simulink model "FinalSimulinkBlock"  (R2017b)
settings: Solver=FixedStepAuto  StartTime=0.0  StopTime=inf  RelTol=1e-3  EnableMultiTasking=on
libraries: simulink_extras x6, simulink x2, embdlinuxlib x2
settings Model: SimulationMode=external  Creator=gtsia  LastModifiedBy=DELL 5548
settings SolverCC: PositivePriorityOrder=on
settings OptimizationCC: PassReuseOutputArgsAs=Individual arguments  MaxStackSize=64
settings DebuggingCC: ParameterTunabilityLossMsg=error
settings HardwareCC: ProdBitPerPointer=32  ProdBitPerSizeT=32  ProdBitPerPtrDiffT=32  ProdLargestAtomicInteger=Long  ProdLargestAtomicFloat=Double  ProdWordSize=32  ProdHWDeviceType=ARM Compatible->ARM Cortex
settings SFSimCC: MATLABDynamicMemAlloc=off
settings RTWCC: SystemTargetFile=ert.tlc  HardwareBoard=Raspberry Pi  TemplateMakefile=ert_default_tmf  GenerateReport=on  Toolchain=GNU GCC Raspberry Pi  IncludeHyperlinkInReport=on  LaunchReport=on  GenerateTraceInfo=on  GenerateTraceReport=on  GenerateTraceReportSl=on  GenerateTraceReportSf=on  GenerateTraceReportEml=on
settings CodeAppCC: ForceParamTrailComments=on  IgnoreCustomStorageClasses=off  OperatorAnnotations=on  SimulinkDataObjDesc=on  SFDataObjDesc=on  InsertBlockDesc=on
settings ERTTargetCC: SupportContinuousTime=on  SupportVariableSizeSignals=on

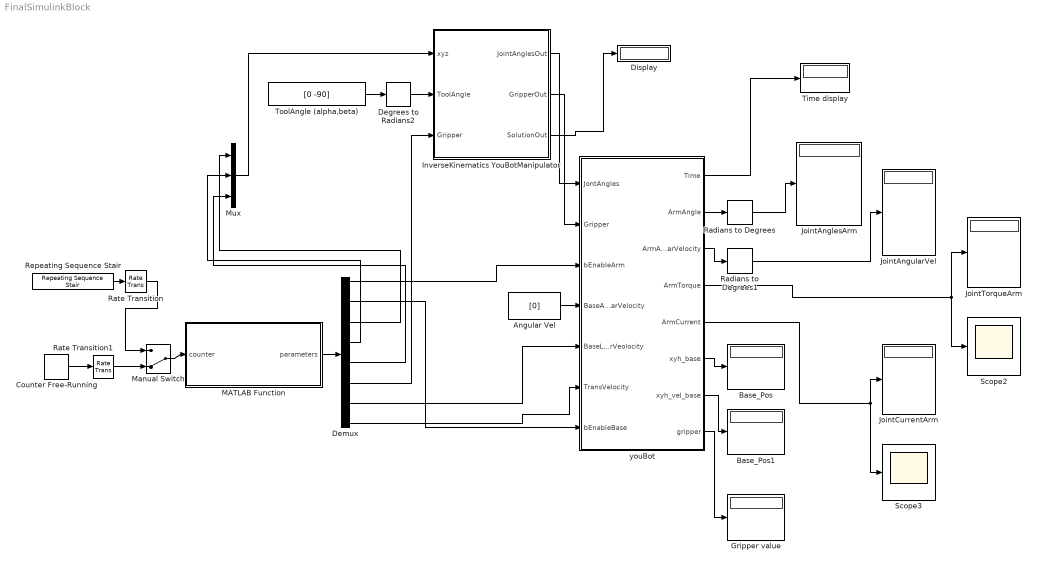
== system FinalSimulinkBlock ==
  Angular Vel : Constant  Value=[0]
  Base_Pos : Display
  Base_Pos1 : Display
  Counter Free-Running : simulink/Sources/Counter Free-Running  NumBits=8  tsamp=6
  Degrees to Radians2 : simulink_extras/Transformations/Degrees to Radians
  Demux : Demux  Outputs=8
  Display : Display
  Gripper value : Display
  InverseKinematics YouBotManipulator : Subsystem
  JointAnglesArm : Display
  JointAngularVel : Display
  JointCurrentArm : Display
  "JointTorqueArm " : Display
  MATLAB Function : MATLAB Function  TreatAsAtomicUnit=on
  Manual Switch : ManualSwitch  CurrentSetting=0
  Mux : Mux  Inputs=3
  Radians to Degrees : simulink_extras/Transformations/Radians to Degrees
  Radians to Degrees1 : simulink_extras/Transformations/Radians to Degrees
  Rate Transition : RateTransition
  Rate Transition1 : RateTransition
  Repeating Sequence Stair : simulink/Sources/Repeating Sequence Stair  OutValues=[0 1 2 3 4 5 6 7 8 9 10 11 11 11 11 11 11].'  tsamp=6  OutMin=[]  OutMax=[]  OutDataTypeStr=double  OutputDataTypeScalingMode=double  OutDataType=fixdt(0,8)  ConRadixGroup=Best Precision: Vector-wise  OutScaling=2^-12
  Scope2 : Scope
  Scope3 : Scope
  Time display : Display
  ToolAngle (alpha,beta) : Constant  Value=[0 -90]
  "youBot " : Subsystem  TreatAsAtomicUnit=on
  wires:
  InverseKinematics YouBotManipulator/2("GripperOut ") -> "youBot "/2(Gripper)
  "youBot "/3(ArmAngularVelocity) -> Radians to Degrees1/1
  "youBot "/1(Time) -> Time display/1
  Radians to Degrees1/1 -> JointAngularVel/1
  Radians to Degrees/1 -> JointAnglesArm/1
  "youBot "/2(ArmAngle) -> Radians to Degrees/1
  "youBot "/6(xyh_base) -> Base_Pos/1
  "youBot "/7(xyh_vel_base) -> Base_Pos1/1
  InverseKinematics YouBotManipulator/1(JointAnglesOut) -> "youBot "/1(JontAngles)
  ToolAngle (alpha,beta)/1 -> Degrees to Radians2/1
  Degrees to Radians2/1 -> InverseKinematics YouBotManipulator/2(ToolAngle)
  Demux/1 -> "youBot "/3(bEnableArm)
  Demux/2 -> "youBot "/7(bEnableBase)
  Demux/3 -> Mux/1
  Demux/4 -> Mux/2
  Demux/5 -> Mux/3
  Demux/6 -> InverseKinematics YouBotManipulator/3(Gripper)
  Demux/7 -> "youBot "/5(BaseLinearVeolocity)
  Demux/8 -> "youBot "/6(TransVelocity)
  Repeating Sequence Stair/1 -> Rate Transition/1
  Manual Switch/1 -> MATLAB Function/1(counter)
  Counter Free-Running/1 -> Rate Transition1/1
  Rate Transition/1 -> Manual Switch/1
  Rate Transition1/1 -> Manual Switch/2
  MATLAB Function/1(parameters) -> Demux/1
  Mux/1 -> InverseKinematics YouBotManipulator/1("xyz ")
  "youBot "/8(gripper) -> Gripper value/1
  InverseKinematics YouBotManipulator/3(SolutionOut) -> Display/1
  Angular Vel/1 -> "youBot "/4("BaseAngularVelocity ")
  "youBot "/4(ArmTorque) -> "JointTorqueArm "/1, Scope2/1
  "youBot "/5(ArmCurrent) -> Scope3/1, JointCurrentArm/1

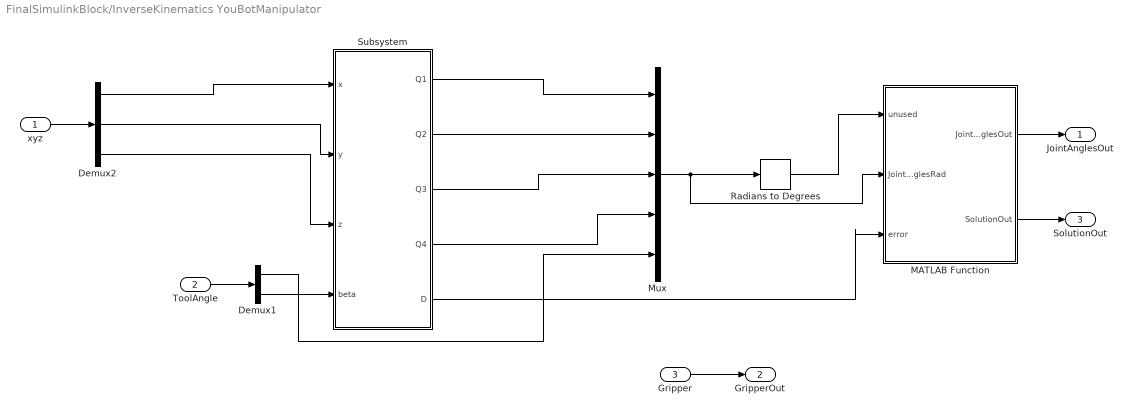
== system FinalSimulinkBlock/InverseKinematics YouBotManipulator ==
  "xyz " : Inport
  ToolAngle : Inport  Port=2
  Gripper : Inport  Port=3
  Demux1 : Demux  Outputs=2
  Demux2 : Demux  Outputs=3
  MATLAB Function : MATLAB Function  TreatAsAtomicUnit=on
  Mux : Mux  Inputs=5
  Radians to Degrees : simulink_extras/Transformations/Radians to Degrees
  Subsystem : Subsystem
  JointAnglesOut : Outport
  "GripperOut " : Outport  Port=2
  SolutionOut : Outport  Port=3
  wires:
  Subsystem/5(D) -> MATLAB Function/3(error)
  Mux/1 -> MATLAB Function/2(JointAnglesRad), Radians to Degrees/1
  Demux1/1 -> Mux/5
  Demux1/2 -> Subsystem/4(beta)
  ToolAngle/1 -> Demux1/1
  "xyz "/1 -> Demux2/1
  Subsystem/3(Q3) -> Mux/3
  Subsystem/2(Q2) -> Mux/2
  Radians to Degrees/1 -> MATLAB Function/1(unused)
  Subsystem/4(Q4) -> Mux/4
  Demux2/1 -> Subsystem/1(x)
  Demux2/2 -> Subsystem/2(y)
  Demux2/3 -> Subsystem/3(z)
  Subsystem/1(Q1) -> Mux/1
  MATLAB Function/2(SolutionOut) -> SolutionOut/1
  MATLAB Function/1(JointAnglesOut) -> JointAnglesOut/1
  Gripper/1 -> "GripperOut "/1

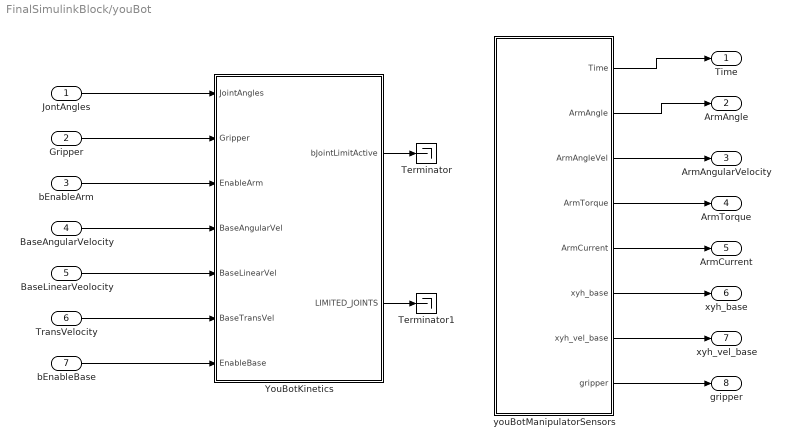
== system FinalSimulinkBlock/youBot  ==
  JontAngles : Inport
  Gripper : Inport  Port=2
  bEnableArm : Inport  Port=3
  "BaseAngularVelocity " : Inport  Port=4
  BaseLinearVeolocity : Inport  Port=5
  TransVelocity : Inport  Port=6
  bEnableBase : Inport  Port=7
  Terminator : Terminator
  Terminator1 : Terminator
  "YouBotKinetics " : Subsystem
  youBotManipulatorSensors : Subsystem
  Time : Outport
  ArmAngle : Outport  Port=2
  ArmAngularVelocity : Outport  Port=3
  ArmTorque : Outport  Port=4
  ArmCurrent : Outport  Port=5
  xyh_base : Outport  Port=6
  xyh_vel_base : Outport  Port=7
  gripper : Outport  Port=8
  wires:
  JontAngles/1 -> "YouBotKinetics "/1(JointAngles)
  Gripper/1 -> "YouBotKinetics "/2(Gripper)
  bEnableArm/1 -> "YouBotKinetics "/3(EnableArm)
  "BaseAngularVelocity "/1 -> "YouBotKinetics "/4(BaseAngularVel)
  BaseLinearVeolocity/1 -> "YouBotKinetics "/5(BaseLinearVel)
  bEnableBase/1 -> "YouBotKinetics "/7("EnableBase ")
  TransVelocity/1 -> "YouBotKinetics "/6(BaseTransVel)
  youBotManipulatorSensors/1(Time) -> Time/1
  youBotManipulatorSensors/2(ArmAngle) -> ArmAngle/1
  youBotManipulatorSensors/3(ArmAngleVel) -> ArmAngularVelocity/1
  youBotManipulatorSensors/4(ArmTorque) -> ArmTorque/1
  youBotManipulatorSensors/5("ArmCurrent ") -> ArmCurrent/1
  youBotManipulatorSensors/6(xyh_base) -> xyh_base/1
  youBotManipulatorSensors/7(xyh_vel_base) -> xyh_vel_base/1
  youBotManipulatorSensors/8(gripper) -> gripper/1
  "YouBotKinetics "/1(bJointLimitActive) -> Terminator/1
  "YouBotKinetics "/2("LIMITED_JOINTS ") -> Terminator1/1

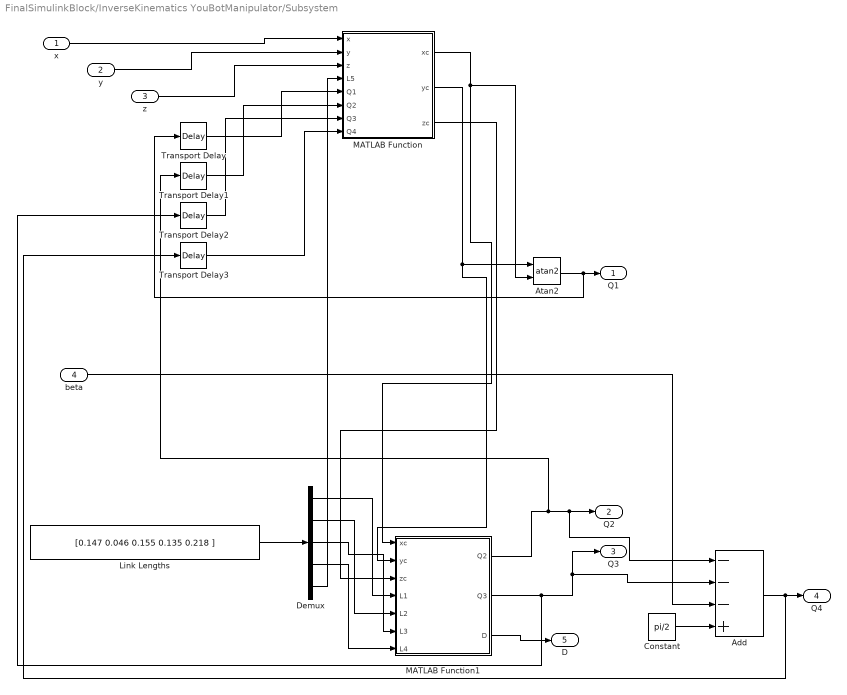
== system FinalSimulinkBlock/InverseKinematics YouBotManipulator/Subsystem ==
  x : Inport
  y : Inport  Port=2
  z : Inport  Port=3
  beta : Inport  Port=4
  Add : Sum  Inputs=---+
  Atan2 : Trigonometry  Operator=atan2
  Constant : Constant  Value=pi/2
  Demux : Demux  Outputs=5
  Link Lengths : Constant  Value=[0.147 0.046 0.155 0.135 0.218 ]
  MATLAB Function : MATLAB Function  TreatAsAtomicUnit=on
  MATLAB Function1 : MATLAB Function  TreatAsAtomicUnit=on
  Transport Delay{,1..3} (4 alike) : TransportDelay
  Q1 : Outport
  Q2 : Outport  Port=2
  Q3 : Outport  Port=3
  Q4 : Outport  Port=4
  D : Outport  Port=5
  wires:
  Demux/2 -> MATLAB Function1/5(L2)
  MATLAB Function/1(xc) -> Atan2/2, MATLAB Function1/1(xc)
  x/1 -> MATLAB Function/1(x)
  z/1 -> MATLAB Function/3(z)
  MATLAB Function1/1(Q2) -> Transport Delay1/1, Q2/1, Add/1
  Add/1 -> Transport Delay3/1, Q4/1
  y/1 -> MATLAB Function/2(y)
  MATLAB Function/3(zc) -> MATLAB Function1/3(zc)
  Link Lengths/1 -> Demux/1
  Demux/4 -> MATLAB Function1/7(L4)
  MATLAB Function1/3(D) -> D/1
  Constant/1 -> Add/4
  MATLAB Function/2(yc) -> Atan2/1, MATLAB Function1/2(yc)
  MATLAB Function1/2(Q3) -> Transport Delay2/1, Q3/1, Add/2
  Demux/3 -> MATLAB Function1/6(L3)
  Demux/1 -> MATLAB Function1/4(L1)
  Atan2/1 -> Transport Delay/1, Q1/1
  beta/1 -> Add/3
  Demux/5 -> MATLAB Function/4(L5)
  Transport Delay/1 -> MATLAB Function/5(Q1)
  Transport Delay1/1 -> MATLAB Function/6(Q2)
  Transport Delay2/1 -> MATLAB Function/7(Q3)
  Transport Delay3/1 -> MATLAB Function/8(Q4)

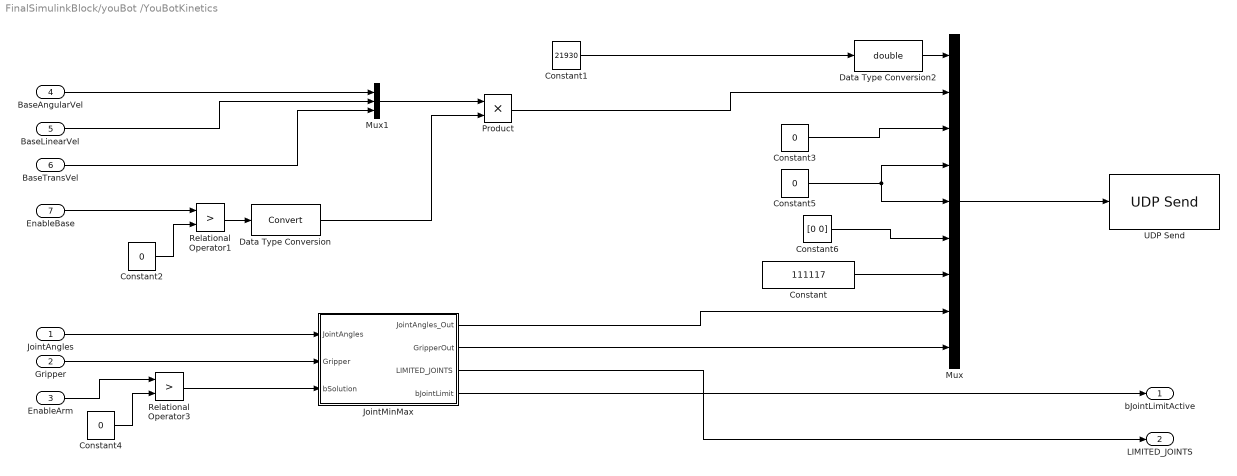
== system FinalSimulinkBlock/youBot /YouBotKinetics  ==
  JointAngles : Inport
  Gripper : Inport  Port=2
  EnableArm : Inport  Port=3
  BaseAngularVel : Inport  Port=4
  BaseLinearVel : Inport  Port=5
  BaseTransVel : Inport  Port=6
  "EnableBase " : Inport  Port=7
  Constant : Constant  Value=111117
  Constant1 : Constant  Value=21930
  Constant{2..5} (4 alike) : Constant  Value=0
  Constant6 : Constant  Value=[0 0]
  Data Type Conversion : DataTypeConversion
  Data Type Conversion2 : DataTypeConversion  OutDataTypeStr=double
  JointMinMax : Subsystem
  Mux : Mux  Inputs=[1 3 1 1 1 2 1 5 1]
  Mux1 : Mux  Inputs=[1 1 1]
  Product : Product
  Relational Operator1 : RelationalOperator  Operator=>  OutDataTypeStr=boolean  RndMeth=Nearest
  Relational Operator3 : RelationalOperator  Operator=>  OutDataTypeStr=boolean  RndMeth=Nearest
  UDP Send : embdlinuxlib/UDP Send  remoteURL='192.168.0.2'  remotePort=25005  localURL='255.255.255.255'  localPortSource=Automatically determine  localPort=-1  sampletime=-1  blockPlatform=Raspberry Pi  separateLengthPort=0
      settings: SourceProductName=Simulink Support Package for Raspberry Pi Hardware  SourceProductBaseCode=RASPPI
  bJointLimitActive : Outport
  "LIMITED_JOINTS " : Outport  Port=2
  wires:
  Mux/1 -> UDP Send/1
  Data Type Conversion2/1 -> Mux/1
  Constant1/1 -> Data Type Conversion2/1
  JointMinMax/1(JointAngles_Out) -> Mux/8
  JointMinMax/2(GripperOut) -> Mux/9
  Gripper/1 -> JointMinMax/2(Gripper)
  JointAngles/1 -> JointMinMax/1(JointAngles)
  JointMinMax/3("LIMITED_JOINTS ") -> "LIMITED_JOINTS "/1
  JointMinMax/4("bJointLimit ") -> bJointLimitActive/1
  Constant/1 -> Mux/7
  BaseAngularVel/1 -> Mux1/1
  BaseLinearVel/1 -> Mux1/2
  BaseTransVel/1 -> Mux1/3
  Constant2/1 -> Relational Operator1/2
  "EnableBase "/1 -> Relational Operator1/1
  Mux1/1 -> Product/1
  Relational Operator1/1 -> Data Type Conversion/1
  Data Type Conversion/1 -> Product/2
  Product/1 -> Mux/2
  Constant4/1 -> Relational Operator3/2
  EnableArm/1 -> Relational Operator3/1
  Constant3/1 -> Mux/3
  Constant5/1 -> Mux/5, Mux/4
  Constant6/1 -> Mux/6
  Relational Operator3/1 -> JointMinMax/3(bSolution)

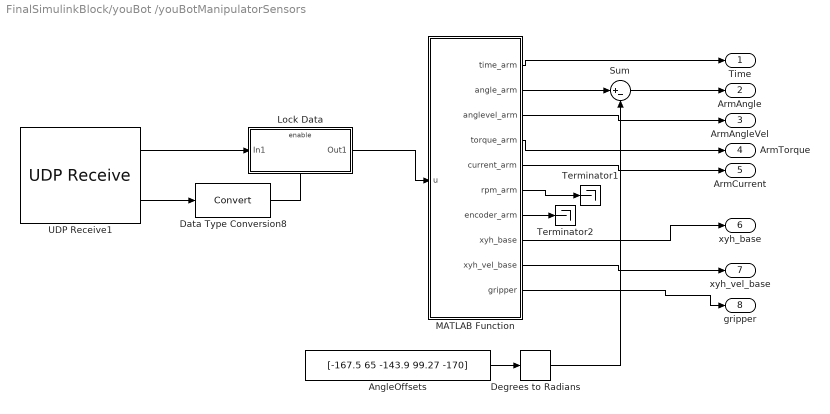
== system FinalSimulinkBlock/youBot /youBotManipulatorSensors ==
  AngleOffsets : Constant  Value=[-167.5 65 -143.9 99.27 -170]
  Data Type Conversion8 : DataTypeConversion
  Degrees to Radians : simulink_extras/Transformations/Degrees to Radians
  Lock Data : Subsystem  TreatAsAtomicUnit=on
  MATLAB Function : MATLAB Function  TreatAsAtomicUnit=on
  Sum : Sum  Inputs=|+-
  Terminator1 : Terminator
  Terminator2 : Terminator
  UDP Receive1 : embdlinuxlib/UDP Receive  localURL='0.0.0.0'  localPort=25611  remoteURL='0.0.0.0'  remotePort=-1  recvBufferSize=8192  signalDatatype=double  dims=62  isVarSize=off  showBlockingTime=off  blockingTime=0  sampletime=0.05  blockPlatform=Raspberry Pi
      settings: SourceProductName=Simulink Support Package for Raspberry Pi Hardware  SourceProductBaseCode=RASPPI
  Time : Outport
  ArmAngle : Outport  Port=2
  ArmAngleVel : Outport  Port=3
  ArmTorque : Outport  Port=4
  "ArmCurrent " : Outport  Port=5
  xyh_base : Outport  Port=6
  xyh_vel_base : Outport  Port=7
  gripper : Outport  Port=8
  wires:
  UDP Receive1/1 -> Lock Data/1(In1)
  Lock Data/1(Out1) -> MATLAB Function/1(u)
  Data Type Conversion8/1 -> Lock Data/Enable
  UDP Receive1/2 -> Data Type Conversion8/1
  MATLAB Function/1(time_arm) -> Time/1
  MATLAB Function/3(anglevel_arm) -> ArmAngleVel/1
  MATLAB Function/4(torque_arm) -> ArmTorque/1
  MATLAB Function/5(current_arm) -> "ArmCurrent "/1
  AngleOffsets/1 -> Degrees to Radians/1
  Sum/1 -> ArmAngle/1
  MATLAB Function/2(angle_arm) -> Sum/1
  Degrees to Radians/1 -> Sum/2
  MATLAB Function/8(xyh_base) -> xyh_base/1
  MATLAB Function/9(xyh_vel_base) -> xyh_vel_base/1
  MATLAB Function/10(gripper) -> gripper/1
  MATLAB Function/6(rpm_arm) -> Terminator1/1
  MATLAB Function/7(encoder_arm) -> Terminator2/1

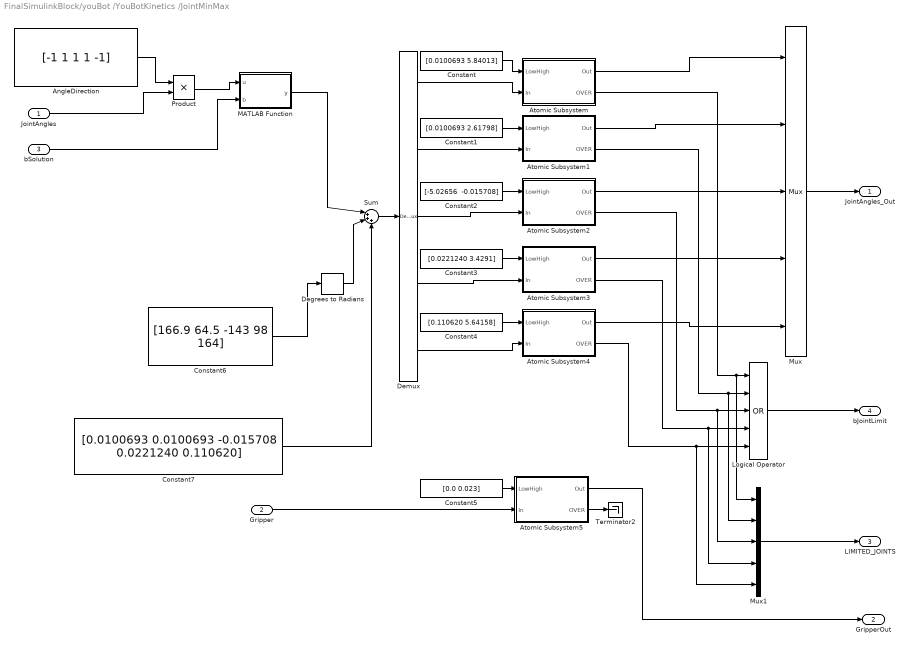
== system FinalSimulinkBlock/youBot /YouBotKinetics /JointMinMax ==
  JointAngles : Inport
  Gripper : Inport  Port=2
  bSolution : Inport  Port=3
  AngleDirection : Constant  Value=[-1 1 1 1 -1]
  Atomic Subsystem : Subsystem  TreatAsAtomicUnit=on
  Atomic Subsystem1 : Subsystem  TreatAsAtomicUnit=on
  Atomic Subsystem2 : Subsystem  TreatAsAtomicUnit=on
  Atomic Subsystem3 : Subsystem  TreatAsAtomicUnit=on
  Atomic Subsystem4 : Subsystem  TreatAsAtomicUnit=on
  Atomic Subsystem5 : Subsystem  TreatAsAtomicUnit=on
  Constant : Constant  Value=[0.0100693 5.84013]
  Constant1 : Constant  Value=[0.0100693 2.61798]
  Constant2 : Constant  Value="[-5.02656  -0.015708]"
  Constant3 : Constant  Value=[0.0221240 3.4291]
  Constant4 : Constant  Value=[0.110620 5.64158]
  Constant5 : Constant  Value=[0.0 0.023]
  Constant6 : Constant  Value=[166.9 64.5 -143 98 164]
  Constant7 : Constant  Value=[0.0100693 0.0100693 -0.015708 0.0221240 0.110620]
  Degrees to Radians : simulink_extras/Transformations/Degrees to Radians
  Demux : Demux  Outputs=[ 1 1 1 1 1]
  Logical Operator : Logic  Operator=OR  Inputs=5  AllPortsSameDT=off  OutDataTypeStr=boolean
  MATLAB Function : MATLAB Function  TreatAsAtomicUnit=on
  Mux : Mux  Inputs=[1 1 1 1 1]
  Mux1 : Mux  Inputs=5
  Product : Product
  Sum : Sum  Inputs=|+++
  Terminator2 : Terminator
  JointAngles_Out : Outport
  GripperOut : Outport  Port=2
  "LIMITED_JOINTS " : Outport  Port=3
  "bJointLimit " : Outport  Port=4
  wires:
  Mux/1 -> JointAngles_Out/1
  Constant/1 -> Atomic Subsystem/1(LowHigh)
  Demux/1 -> Atomic Subsystem/2(In)
  Constant4/1 -> Atomic Subsystem4/1(LowHigh)
  Constant3/1 -> Atomic Subsystem3/1(LowHigh)
  Constant2/1 -> Atomic Subsystem2/1(LowHigh)
  Constant1/1 -> Atomic Subsystem1/1(LowHigh)
  Demux/2 -> Atomic Subsystem1/2(In)
  Atomic Subsystem/1(Out) -> Mux/1
  Demux/4 -> Atomic Subsystem3/2(In)
  Demux/3 -> Atomic Subsystem2/2(In)
  Atomic Subsystem1/1(Out) -> Mux/2
  Atomic Subsystem2/1(Out) -> Mux/3
  Atomic Subsystem3/1(Out) -> Mux/4
  Demux/5 -> Atomic Subsystem4/2(In)
  Atomic Subsystem4/1(Out) -> Mux/5
  Atomic Subsystem/2(OVER) -> Mux1/1, Logical Operator/1
  Atomic Subsystem1/2(OVER) -> Mux1/2, Logical Operator/2
  Atomic Subsystem2/2(OVER) -> Mux1/3, Logical Operator/3
  Atomic Subsystem3/2(OVER) -> Mux1/4, Logical Operator/4
  Atomic Subsystem4/2(OVER) -> Mux1/5, Logical Operator/5
  Mux1/1 -> "LIMITED_JOINTS "/1
  Gripper/1 -> Atomic Subsystem5/2(In)
  Constant5/1 -> Atomic Subsystem5/1(LowHigh)
  Sum/1 -> Demux/1
  Degrees to Radians/1 -> Sum/2
  Constant6/1 -> Degrees to Radians/1
  Constant7/1 -> Sum/3
  JointAngles/1 -> Product/2
  Logical Operator/1 -> "bJointLimit "/1
  Atomic Subsystem5/1(Out) -> GripperOut/1
  Atomic Subsystem5/2(OVER) -> Terminator2/1
  AngleDirection/1 -> Product/1
  bSolution/1 -> MATLAB Function/2(b)
  Product/1 -> MATLAB Function/1(u)
  MATLAB Function/1(y) -> Sum/1

== system FinalSimulinkBlock/youBot /youBotManipulatorSensors/Lock Data ==
  In1 : Inport
  Enable : EnablePort
  Out1 : Outport
  wires:
  In1/1 -> Out1/1

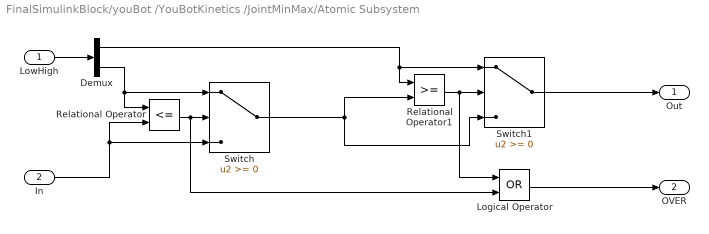
== system FinalSimulinkBlock/youBot /YouBotKinetics /JointMinMax/Atomic Subsystem ==
  LowHigh : Inport
  In : Inport  Port=2
  Demux : Demux  Outputs=2
  Logical Operator : Logic  Operator=OR  AllPortsSameDT=off  OutDataTypeStr=boolean
  Relational Operator : RelationalOperator  Operator=<=  OutDataTypeStr=boolean  RndMeth=Nearest
  Relational Operator1 : RelationalOperator  OutDataTypeStr=boolean  RndMeth=Nearest
  Switch : Switch
  Switch1 : Switch
  Out : Outport
  OVER : Outport  Port=2
  wires:
  In/1 -> Relational Operator/2, Switch/3
  LowHigh/1 -> Demux/1
  Relational Operator/1 -> Logical Operator/2, Switch/2
  Demux/2 -> Switch/1, Relational Operator/1
  Switch/1 -> Switch1/3, Relational Operator1/2
  Switch1/1 -> Out/1
  Relational Operator1/1 -> Logical Operator/1, Switch1/2
  Demux/1 -> Switch1/1, Relational Operator1/1
  Logical Operator/1 -> OVER/1

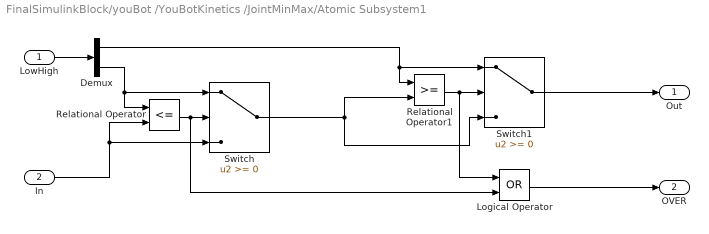
== system FinalSimulinkBlock/youBot /YouBotKinetics /JointMinMax/Atomic Subsystem1 ==
  LowHigh : Inport
  In : Inport  Port=2
  Demux : Demux  Outputs=2
  Logical Operator : Logic  Operator=OR  AllPortsSameDT=off  OutDataTypeStr=boolean
  Relational Operator : RelationalOperator  Operator=<=  OutDataTypeStr=boolean  RndMeth=Nearest
  Relational Operator1 : RelationalOperator  OutDataTypeStr=boolean  RndMeth=Nearest
  Switch : Switch
  Switch1 : Switch
  Out : Outport
  OVER : Outport  Port=2
  wires:
  In/1 -> Relational Operator/2, Switch/3
  LowHigh/1 -> Demux/1
  Relational Operator/1 -> Logical Operator/2, Switch/2
  Demux/2 -> Switch/1, Relational Operator/1
  Switch/1 -> Switch1/3, Relational Operator1/2
  Switch1/1 -> Out/1
  Relational Operator1/1 -> Logical Operator/1, Switch1/2
  Demux/1 -> Switch1/1, Relational Operator1/1
  Logical Operator/1 -> OVER/1

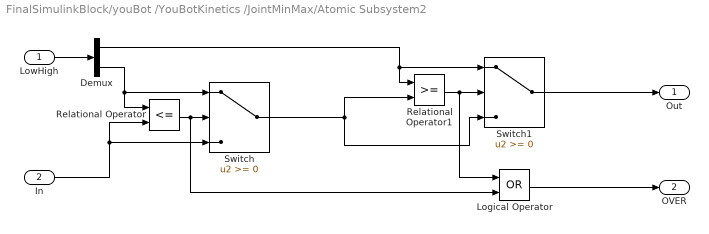
== system FinalSimulinkBlock/youBot /YouBotKinetics /JointMinMax/Atomic Subsystem2 ==
  LowHigh : Inport
  In : Inport  Port=2
  Demux : Demux  Outputs=2
  Logical Operator : Logic  Operator=OR  AllPortsSameDT=off  OutDataTypeStr=boolean
  Relational Operator : RelationalOperator  Operator=<=  OutDataTypeStr=boolean  RndMeth=Nearest
  Relational Operator1 : RelationalOperator  OutDataTypeStr=boolean  RndMeth=Nearest
  Switch : Switch
  Switch1 : Switch
  Out : Outport
  OVER : Outport  Port=2
  wires:
  In/1 -> Relational Operator/2, Switch/3
  LowHigh/1 -> Demux/1
  Relational Operator/1 -> Logical Operator/2, Switch/2
  Demux/2 -> Switch/1, Relational Operator/1
  Switch/1 -> Switch1/3, Relational Operator1/2
  Switch1/1 -> Out/1
  Relational Operator1/1 -> Logical Operator/1, Switch1/2
  Demux/1 -> Switch1/1, Relational Operator1/1
  Logical Operator/1 -> OVER/1

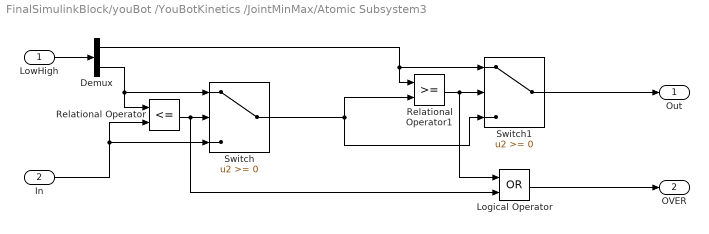
== system FinalSimulinkBlock/youBot /YouBotKinetics /JointMinMax/Atomic Subsystem3 ==
  LowHigh : Inport
  In : Inport  Port=2
  Demux : Demux  Outputs=2
  Logical Operator : Logic  Operator=OR  AllPortsSameDT=off  OutDataTypeStr=boolean
  Relational Operator : RelationalOperator  Operator=<=  OutDataTypeStr=boolean  RndMeth=Nearest
  Relational Operator1 : RelationalOperator  OutDataTypeStr=boolean  RndMeth=Nearest
  Switch : Switch
  Switch1 : Switch
  Out : Outport
  OVER : Outport  Port=2
  wires:
  In/1 -> Relational Operator/2, Switch/3
  LowHigh/1 -> Demux/1
  Relational Operator/1 -> Logical Operator/2, Switch/2
  Demux/2 -> Switch/1, Relational Operator/1
  Switch/1 -> Switch1/3, Relational Operator1/2
  Switch1/1 -> Out/1
  Relational Operator1/1 -> Logical Operator/1, Switch1/2
  Demux/1 -> Switch1/1, Relational Operator1/1
  Logical Operator/1 -> OVER/1

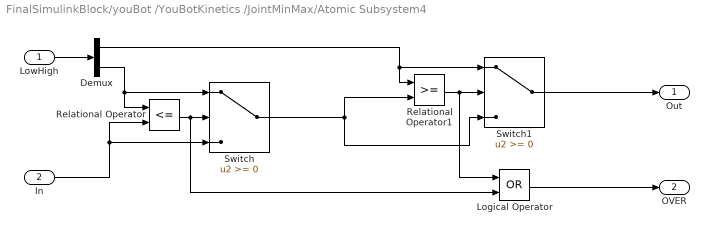
== system FinalSimulinkBlock/youBot /YouBotKinetics /JointMinMax/Atomic Subsystem4 ==
  LowHigh : Inport
  In : Inport  Port=2
  Demux : Demux  Outputs=2
  Logical Operator : Logic  Operator=OR  AllPortsSameDT=off  OutDataTypeStr=boolean
  Relational Operator : RelationalOperator  Operator=<=  OutDataTypeStr=boolean  RndMeth=Nearest
  Relational Operator1 : RelationalOperator  OutDataTypeStr=boolean  RndMeth=Nearest
  Switch : Switch
  Switch1 : Switch
  Out : Outport
  OVER : Outport  Port=2
  wires:
  In/1 -> Relational Operator/2, Switch/3
  LowHigh/1 -> Demux/1
  Relational Operator/1 -> Logical Operator/2, Switch/2
  Demux/2 -> Switch/1, Relational Operator/1
  Switch/1 -> Switch1/3, Relational Operator1/2
  Switch1/1 -> Out/1
  Relational Operator1/1 -> Logical Operator/1, Switch1/2
  Demux/1 -> Switch1/1, Relational Operator1/1
  Logical Operator/1 -> OVER/1

== system FinalSimulinkBlock/youBot /YouBotKinetics /JointMinMax/Atomic Subsystem5 ==
  LowHigh : Inport
  In : Inport  Port=2
  Demux : Demux  Outputs=2
  Logical Operator : Logic  Operator=OR  AllPortsSameDT=off  OutDataTypeStr=boolean
  Relational Operator : RelationalOperator  Operator=<=  OutDataTypeStr=boolean  RndMeth=Nearest
  Relational Operator1 : RelationalOperator  OutDataTypeStr=boolean  RndMeth=Nearest
  Switch : Switch
  Switch1 : Switch
  Out : Outport
  OVER : Outport  Port=2
  wires:
  In/1 -> Relational Operator/2, Switch/3
  LowHigh/1 -> Demux/1
  Relational Operator/1 -> Logical Operator/2, Switch/2
  Demux/2 -> Switch/1, Relational Operator/1
  Switch/1 -> Switch1/3, Relational Operator1/2
  Switch1/1 -> Out/1
  Relational Operator1/1 -> Logical Operator/1, Switch1/2
  Demux/1 -> Switch1/1, Relational Operator1/1
  Logical Operator/1 -> OVER/1

== matlab function FinalSimulinkBlock/MATLAB Function ==
  data: counter input; parameters output
function parameters = Sequence(counter)
    %This function extracts the desired parameters in a vector for each
    %evaluated step 
    %parameters = [enablearm enablebase x y z gripper linear transversal]
    
    if counter == 0
        parameters = [1 0 0.3 0 -0.08 0.01 0 0]; % go to pick up position (12 o'clock)
    elseif counter == 1
        parameters = [1 0 0.3 0 -0.08 0 0 0]; % close gripper to grab the cude
    elseif counter == 2
        parameters = [1 0 -0.27 -0.01 0.11 0 0 0]; % go to router position
    elseif counter == 3
        parameters = [1 0 -0.27 -0.01 0.11 0 0 0]; %go to router position
    elseif counter == 4
        parameters = [1 0 -0.27 -0.01 0.11 0.01 0 0]; %go to router position
    elseif counter == 5
        parameters = [1 0 -0.27 -0.01 0.11 0.01 0 0]; % %open gripper to router position to leave the cube
    elseif counter == 6
        parameters = [1 0 1 1 1 0.01 0 0]; %go to default position
    elseif counter == 7
        parameters = [0 1 0 0.3 0.5 0.01 0 0.1666]; %start moving with linear velocity
    elseif counter == 8
        parameters = [0 1 0 0.3 0.5 0.01 0 0.1666]; %start moving with transversal velocity
    elseif counter == 9
        parameters = [1 0 -0.25 -0.01 0.13 0.01 0 0]; %go to router (n-1) position
    elseif counter == 10
       parameters = [1 0 -0.25 -0.01 0.13 0.01 0 0]; %go to router (n-1) position
    elseif counter == 11
        parameters = [1 0 -0.25 -0.01 0.13 0.01 0 0]; %go to router (n-1) position
    elseif counter == 12
        parameters = [1 0 -0.28 -0.01 0.095 0.01 0 0]; %go to cube position
    elseif counter == 13
        parameters = [1 0 -0.28 -0.01 0.095 0 0 0]; % close gripper and grab the cube
    elseif counter == 14
        parameters = [1 0 0 0.18 0.18 0 0 0]; %go to desired position
    elseif counter == 15
        parameters = [1 0 0 0.18 0.18 0 0 0]; %go to desired position
    elseif counter == 16
        parameters = [1 0 0 0.18 0.18 0 0 0]; %go to desired position
    elseif counter == 17
        parameters = [1 0 0 0.18 0.18 0 0 0]; %go to desired position
    elseif counter == 18
        parameters = [1 0 0 0.18 0.18 0.01 0 0]; %open gripper and leave cube to desired position
    elseif counter == 19
        parameters = [1 0 1 1 1 0.01 0 0]; %return to default position
    else
        parameters = [0 0 0 0 0 0 0 0]; %do nothing
    end
end

== matlab function FinalSimulinkBlock/youBot /YouBotKinetics /JointMinMax/MATLAB Function ==
  data: u input; y output; b input
function y = fcn(u,b)
if(b>0)
    y = u;
else 
    y=0*u;
end

== matlab function FinalSimulinkBlock/youBot /youBotManipulatorSensors/MATLAB Function ==
  data: u input; time_arm output; angle_arm output; anglevel_arm output; torque_arm output; current_arm output; rpm_arm output; encoder_arm output; xyh_base output; xyh_vel_base output; gripper output
function [time_arm,angle_arm, anglevel_arm, torque_arm, current_arm, rpm_arm, encoder_arm ,xyh_base,xyh_vel_base, gripper] = decodeYouBotSensorPacket(u)
    n=(0:4)*10+1;
    time_arm=u(n);
    angle_arm=u(n+1).*[-1 1 1 1 -1]';
    current_arm=u(n+2);
    torque_arm=u(n+3);
    anglevel_arm=u(n+4).*[-1 1 1 1 -1]';
    encoder_arm=u(n+5);
    rpm_arm=u(n+6);
    xyh_base=u(52:54);
    xyh_vel_base=u(55:57);
    gripper=u(61);

== matlab function FinalSimulinkBlock/InverseKinematics YouBotManipulator/MATLAB Function ==
  data: unused input; JointAnglesOut output; JointAnglesRad input; error input; SolutionOut output
function [JointAnglesOut,SolutionOut] = out(~, JointAnglesRad, error)


    if error>1
        SolutionOut = 0;
        JointAnglesOut = 0*(JointAnglesRad);
    else
        SolutionOut = 1;
        JointAnglesOut = JointAnglesRad;

end

== matlab function FinalSimulinkBlock/InverseKinematics YouBotManipulator/Subsystem/MATLAB Function ==
  data: x input; xc output; y input; z input; L5 input; Q1 input; Q2 input; Q3 input; Q4 input; yc output; zc output
function [xc,yc,zc] = Oc(x,y,z,L5,Q1,Q2,Q3,Q4)

%forward kinematics
r13 = cos(Q1)*sin(Q2+Q3+Q4);
r23 = sin(Q1)*sin(Q2+Q3+Q4);
r33 = cos(Q2+Q3+Q4);

%position of Oc

xc = x - L5*r13;
yc = y - L5*r23;
zc = z - L5*r33;

end

== matlab function FinalSimulinkBlock/InverseKinematics YouBotManipulator/Subsystem/MATLAB Function1 ==
  data: xc input; Q2 output; yc input; zc input; L1 input; L2 input; L3 input; L4 input; Q3 output; D output
function [Q2,Q3,D] = ang(xc,yc,zc,L1,L2,L3,L4)

D = ((xc.^2 + yc.^2 - 2*sqrt(xc.^2 + yc.^2)*L2 + L2.^2)+(zc-L1).^2 - L3.^2-L4.^2)/(2*L3*L4);

    if D>1
        Q3 = 0;
        Q2 = 0;
    else
        Q3 = atan2(sqrt(1-D.^2),D);
        Q2 = atan2((sqrt(xc.^2+yc.^2)-L2),zc-L1) - atan2(L4*sin(Q3),L3+L4*cos(Q3));
    end
end
